simulink model "DatosPaso1R16"  (R2022b)
settings: Solver=ode45  StartTime=0.0  StopTime=20  RelTol=1e-3  EnableMultiTasking=on
settings Model: Creator=Helbert  LastModifiedBy=PC-LUISMIGUEL
settings SolverCC: AlgebraicLoopSolver=TrustRegion
settings DataIOCC: LimitDataPoints=on  SaveFormat=Array  SignalLoggingSaveFormat=ModelDataLogs  ReturnWorkspaceOutputs=off
settings OptimizationCC: InitFltsAndDblsToZero=on  LifeSpan=inf
settings DebuggingCC: SaveWithParameterizedLinksMsg=none  UnderspecifiedInitializationDetection=Classic  MergeDetectMultiDrivingBlocksExec=none  SignalResolutionControl=TryResolveAllWithWarning  SolverPrmCheckMsg=warning  MultiTaskDSMMsg=warning  MultiTaskCondExecSysMsg=none  UnconnectedInputMsg=warning  UnconnectedOutputMsg=warning  UnconnectedLineMsg=warning  SFUnexpectedBacktrackingDiag=warning  SFNoUnconditionalDefaultTransitionDiag=warning  SFExecutionAtInitializationDiag=none  SFMachineParentedDataDiag=warning  ArithmeticOperatorsInVariantConditions=warning
settings HardwareCC: ProdBitPerPointer=32  ProdBitPerSizeT=32  ProdBitPerPtrDiffT=32  ProdLargestAtomicFloat=None  ProdIntDivRoundTo=Undefined  ProdEndianess=Unspecified  ProdWordSize=32  ProdHWDeviceType=32-bit Generic
settings ModelReferenceCC: EnableRefExpFcnMdlSchedulingChecks=on  PropagateSignalLabelsOutOfModel=off
settings SFSimCC: SimUseLocalCustomCode=off  CustomCodeUndefinedFunction=UseInterfaceOnly
settings RTWCC: RTWUseLocalCustomCode=off
settings CodeAppCC: StateflowObjectComments=on
settings GRTTargetCC: TargetFcnLib=ansi_tfl_tmw.mat  TargetLangStandard=C89/C90 (ANSI)  CombineOutputUpdateFcns=off  GRTInterface=on
settings ConfigComp: CovMetricSettings=dw  CovSaveCumulativeToWorkspaceVar=on  CovSaveSingleToWorkspaceVar=on  CovExternalEMLEnable=off

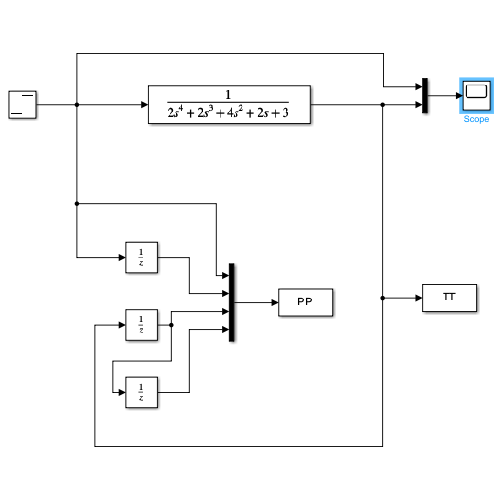
[thumbnail: Simulink's stored preview of the top-level diagram]
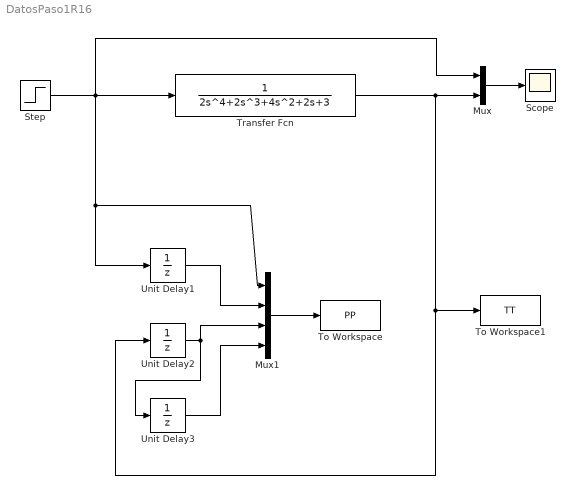
== system DatosPaso1R16 ==
  Mux : Mux  Inputs=2
  Mux1 : Mux
  Scope : Scope
  Step : Step  Time=0  SampleTime=10
  To Workspace : ToWorkspace  VariableName=PP  SampleTime=0.1
  To Workspace1 : ToWorkspace  VariableName=TT  SampleTime=0.1
  Transfer Fcn : TransferFcn  Denominator=[2 2 4 2 3]
  Unit Delay1 : UnitDelay  SampleTime=0.1  HasFrameUpgradeWarning=on
  Unit Delay2 : UnitDelay  SampleTime=0.1  HasFrameUpgradeWarning=on
  Unit Delay3 : UnitDelay  SampleTime=0.1  HasFrameUpgradeWarning=on
  wires:
  Transfer Fcn/1 -> To Workspace1/1, Unit Delay2/1, Mux/2
  Unit Delay2/1 -> Unit Delay3/1, Mux1/3
  Mux1/1 -> To Workspace/1
  Unit Delay1/1 -> Mux1/2
  Unit Delay3/1 -> Mux1/4
  Step/1 -> Unit Delay1/1, Mux1/1, Transfer Fcn/1, Mux/1
  Mux/1 -> Scope/1
